simulink library "INT_Tra_GearInfo"  (R2016b)
settings: Solver=VariableStepAuto  StartTime=0.0  StopTime=10.0  RelTol=1e-3
settings Model: Creator=bianxuyin  LastModifiedBy=bianxuyin

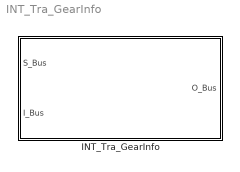
== system INT_Tra_GearInfo ==
  INT_Tra_GearInfo : Subsystem

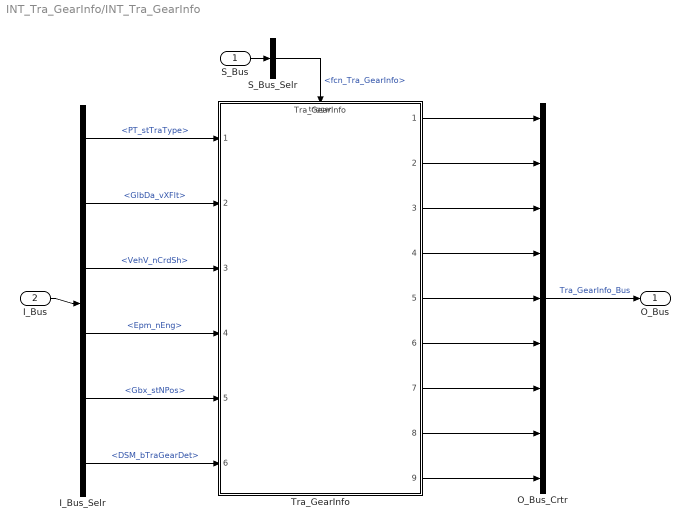
== system INT_Tra_GearInfo/INT_Tra_GearInfo ==
  S_Bus : Inport
  I_Bus : Inport  Port=2
  I_Bus_Selr : BusSelector  OutputSignals=PT_stTraType,GlbDa_vXFlt,VehV_nCrdSh,Epm_nEng,Gbx_stNPos,DSM_bTraGearDet
  O_Bus_Crtr : BusCreator  Inputs=9
  S_Bus_Selr : BusSelector  OutputSignals=fcn_Tra_GearInfo
  Tra_GearInfo : ModelReference  ModelNameDialog=Tra_GearInfo  SimulationMode=Normal  ModelReferenceVersion=1.64  TriggerPortName=function  TriggerPortTriggerType=function-call  TriggerPortStatesWhenEnabling=held
  O_Bus : Outport
  wires:
  S_Bus_Selr/1 -> Tra_GearInfo/Trigger  "<fcn_Tra_GearInfo>"
  S_Bus/1 -> S_Bus_Selr/1
  I_Bus/1 -> I_Bus_Selr/1
  I_Bus_Selr/1 -> Tra_GearInfo/1  "<PT_stTraType>"
  I_Bus_Selr/2 -> Tra_GearInfo/2  "<GlbDa_vXFlt>"
  I_Bus_Selr/3 -> Tra_GearInfo/3  "<VehV_nCrdSh>"
  I_Bus_Selr/4 -> Tra_GearInfo/4  "<Epm_nEng>"
  I_Bus_Selr/5 -> Tra_GearInfo/5  "<Gbx_stNPos>"
  I_Bus_Selr/6 -> Tra_GearInfo/6  "<DSM_bTraGearDet>"
  O_Bus_Crtr/1 -> O_Bus/1  "Tra_GearInfo_Bus"
  Tra_GearInfo/1 -> O_Bus_Crtr/1
  Tra_GearInfo/2 -> O_Bus_Crtr/2
  Tra_GearInfo/3 -> O_Bus_Crtr/3
  Tra_GearInfo/4 -> O_Bus_Crtr/4
  Tra_GearInfo/5 -> O_Bus_Crtr/5
  Tra_GearInfo/6 -> O_Bus_Crtr/6
  Tra_GearInfo/7 -> O_Bus_Crtr/7
  Tra_GearInfo/8 -> O_Bus_Crtr/8
  Tra_GearInfo/9 -> O_Bus_Crtr/9
